simulink model "Ej_1"  (R2023b)
settings: Solver=VariableStepAuto  StartTime=0.0  StopTime=30  MaxStep=1e-4  RelTol=1e-3
values from neighbouring files (symbols this model uses):
  a = 200    [Parametros.m]
  b = 10000    [Parametros.m]
  g = 9.82    [Parametros.m]
  m = 1000    [Parametros.m]
libraries: SignalEditorBlockLib x1
settings Model: Creator=MSI  LastModifiedBy=MSI

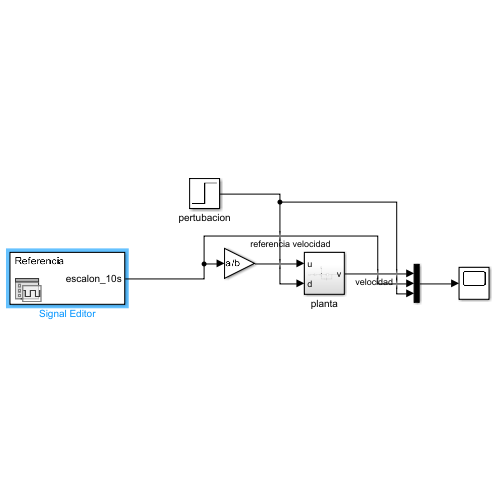
[thumbnail: Simulink's stored preview of the top-level diagram]
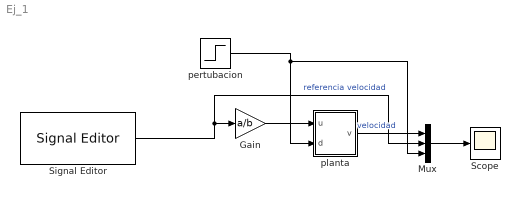
== system Ej_1 ==
  Gain : Gain  Gain=a/b
  Mux : Mux  Inputs=3
  Scope : Scope
  Signal Editor : SignalEditorBlockLib/Signal Editor  FileName=escalon.mat  ActiveScenario=Referencia  ActiveSignal=escalon_10s  IsBus=off  OutputBusObjectStr=Bus: BusObject  SampleTime=0  Interpolate=off  ZeroCross=off  OutputAfterFinalValue=Setting to zero  Unit=inherit  PreserveSignalName=on  ApplySigPropsToAllScenarios=on  ApplySigPropsToAllSignals=off
  pertubacion : Step  Time=5  After=g*sin(2*pi/180)  SampleTime=0
  planta : Subsystem
  wires:
  Gain/1 -> planta/1(u)
  planta/1(v) -> Mux/1  "velocidad"
  Mux/1 -> Scope/1
  Signal Editor/1 -> Gain/1, Mux/2  "referencia velocidad"
  pertubacion/1 -> Mux/3, planta/2(d)

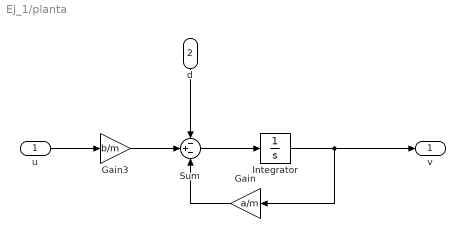
== system Ej_1/planta ==
  u : Inport
  d : Inport  Port=2
  Gain : Gain  Gain=a/m
  Gain3 : Gain  Gain=b/m
  Integrator : Integrator
  Sum : Sum  Inputs=-+-
  v : Outport
  wires:
  Integrator/1 -> v/1, Gain/1
  Gain/1 -> Sum/3
  Gain3/1 -> Sum/2
  d/1 -> Sum/1
  u/1 -> Gain3/1
  Sum/1 -> Integrator/1
